simulink model "Robot_Project"  (R2025b)
settings: Solver=FixedStepDiscrete  StartTime=0.0  StopTime=10  FixedStep=0.01  RelTol=1e-3
model workspace (MAT data in the model file):
  Left_gain_calibration = 2.30921052632
  Right_gain_calibration = 1.47057847023
settings Model: Creator=Ahmed  LastModifiedBy=ENJAZ

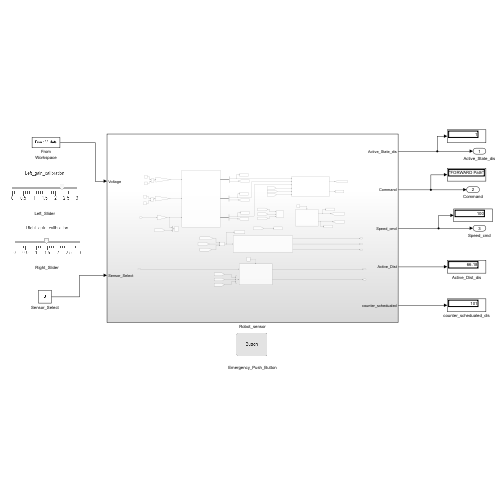
[thumbnail: Simulink's stored preview of the top-level diagram]
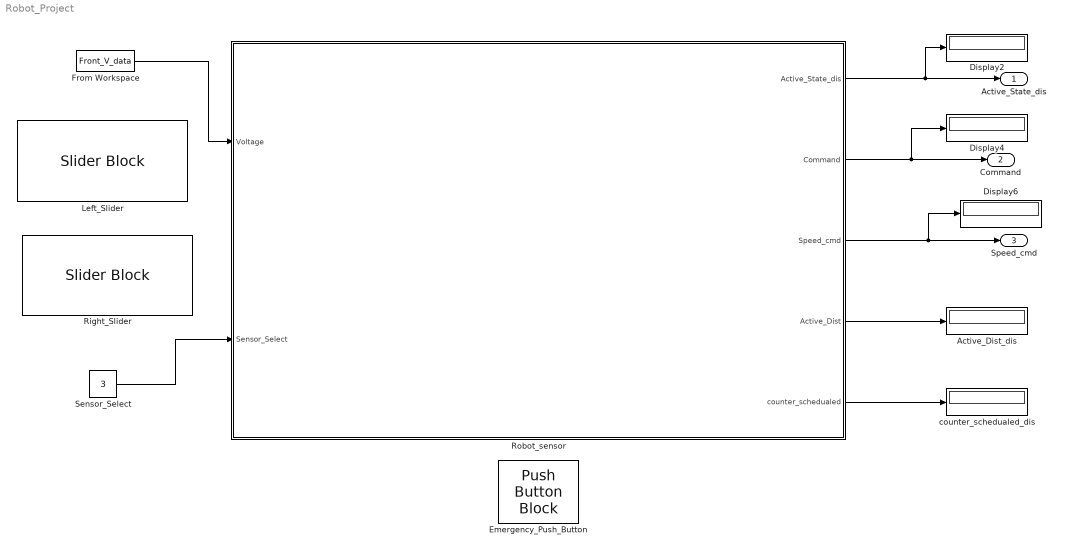
== system Robot_Project ==
  Active_Dist_dis : Display
  Display2 : Display
  Display4 : Display
  Display6 : Display
  Emergency_Push_Button : PushButtonBlock  ButtonType=Latch  IconOnColor=[0.0, 0.39215686274509803, 0.0]  IconOffColor=[0.0, 1.0, 0.0]  OffValue=0.000000
  From Workspace : FromWorkspace  VariableName=Front_V_data
  Left_Slider : SliderBlock  ScaleMax=3
  Right_Slider : SliderBlock  ScaleMax=3
  Robot_sensor : Subsystem
  Sensor_Select : Constant  Value=3
  counter_schedualed_dis : Display
  Active_State_dis : Outport
  Command : Outport  Port=2
  Speed_cmd : Outport  Port=3
  wires:
  Robot_sensor/2(Command) -> Command/1, Display4/1
  Robot_sensor/3(Speed_cmd) -> Display6/1, Speed_cmd/1
  From Workspace/1 -> Robot_sensor/1(Voltage)
  Sensor_Select/1 -> Robot_sensor/2(Sensor_Select)
  Robot_sensor/4(Active_Dist) -> Active_Dist_dis/1
  Robot_sensor/5(counter_schedualed) -> counter_schedualed_dis/1
  Robot_sensor/1(Active_State_dis) -> Active_State_dis/1, Display2/1

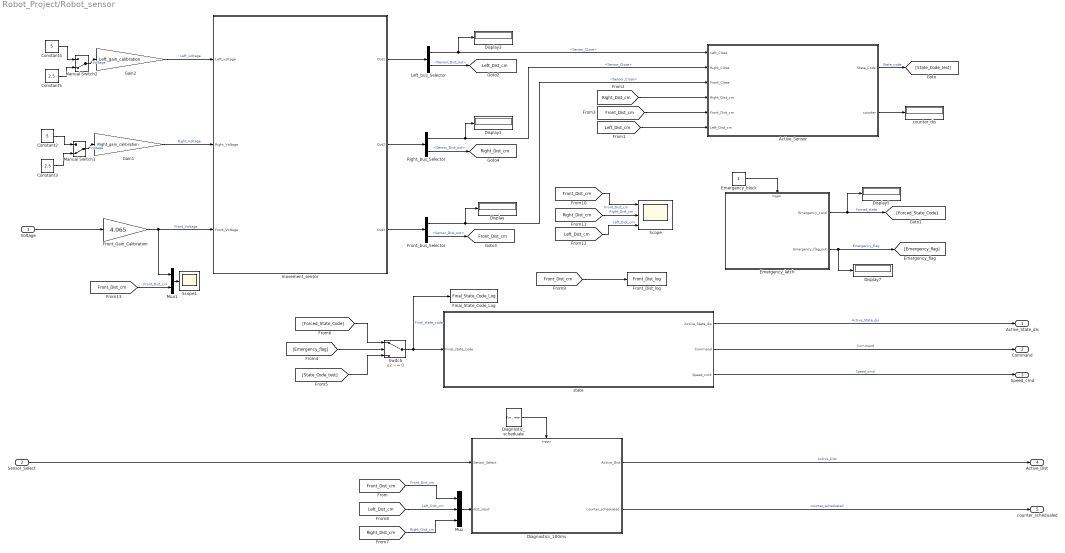
== system Robot_Project/Robot_sensor ==
  Voltage : Inport
  Sensor_Select : Inport  Port=2
  Active_Sensor : Subsystem
  Constant2 : Constant  Value=5
  Constant3 : Constant  Value=2.5
  Constant4 : Constant  Value=5
  Constant5 : Constant  Value=2.5
  Diagnostic_scheduale : FunctionCallGenerator  SampleTime=0.1
  Diagnostics_100ms : Subsystem  TreatAsAtomicUnit=on
  Display{,1,3,5,7} (5 alike) : Display
  Emergency_block : Constant
  Emergency_latch : Subsystem  TreatAsAtomicUnit=on
  Final_State_Code_Log : ToWorkspace  VariableName=Final_State_Code_Log  SaveFormat=Timeseries  SampleTime=-1
  Front_Dist_log : ToWorkspace  VariableName=Front_Dist_log  SaveFormat=Structure With Time  SampleTime=-1
  Front_Gain_Calibration : Gain  Gain=4.065
  Front_bus_Selector : BusSelector  OutputSignals=Sensor_Close,Sensor_Dist_out
  Gain1 : Gain  Gain=Right_gain_calibration
  Gain2 : Gain  Gain=Left_gain_calibration
  Left_bus_Selector : BusSelector  OutputSignals=Sensor_Close,Sensor_Dist_out
  Manual Switch1 : ManualSwitch  CurrentSetting=0
  Manual Switch2 : ManualSwitch  CurrentSetting=0
  Mux : Mux  Inputs=3
  Mux1 : Mux  Inputs=2
  Right_bus_Selector : BusSelector  OutputSignals=Sensor_Close,Sensor_Dist_out
  Scope : Scope  NumInputPorts=3
      settings: ActiveDisplayYMinimum=-1  ActiveDisplayYMaximum=1
  Scope1 : Scope
      settings: ActiveDisplayYMinimum=-43.187499999999993  ActiveDisplayYMaximum=393.6875
  Switch : Switch  Criteria=u2 ~= 0  SaturateOnIntegerOverflow=off  InputSameDT=off
  counter_dis : Display
  movement_sensor : Subsystem
  state : Subsystem
  Active_State_dis : Outport
  Command : Outport  Port=2
  Speed_cmd : Outport  Port=3
  Active_Dist : Outport  Port=4
  counter_schedualed : Outport  Port=5
  tag scope: Front_Dist_cm=global, Left_Dist_cm=global, Right_Dist_cm=global
  wires:
  Left_bus_Selector/1 -> Display3/1, Active_Sensor/1(Left_Close)  "<Sensor_Close>"
  state/1(Active_State_dis) -> Active_State_dis/1  "Active_State_dis"
  Manual Switch2/1 -> Gain2/1  "Voltage"
  Emergency_latch/1(Emergency_cond) -> Display5/1, [Forced_State_Code]  "forced_state"
  Manual Switch1/1 -> Gain1/1  "Voltage"
  [Right_Dist_cm] -> Mux/3  "Right_Dist_cm"
  Diagnostics_100ms/1(Active_Dist) -> Active_Dist/1  "Active_Dist"
  [Front_Dist_cm] -> Front_Dist_log/1
  Right_bus_Selector/1 -> Active_Sensor/2(Right_Close), Display1/1  "<Sensor_Close>"
  Diagnostic_scheduale/1 -> Diagnostics_100ms/Trigger
  [Front_Dist_cm] -> Active_Sensor/5(Front_Dist_cm)
  [State_Code_test] -> Switch/3
  Constant4/1 -> Manual Switch2/1
  [Forced_State_Code] -> Switch/1
  Front_Gain_Calibration/1 -> movement_sensor/3(Front_Voltage), Mux1/1  "Front_Voltage"
  state/2(Command) -> Command/1  "Command"
  Sensor_Select/1 -> Diagnostics_100ms/1(Sensor_Select)
  Front_bus_Selector/1 -> Active_Sensor/3(Front_Close), Display/1  "<Sensor_Close>"
  [Left_Dist_cm] -> Mux/2  "Left_Dist_cm"
  [Front_Dist_cm] -> Mux1/2  "Front_Dist_cm"
  Active_Sensor/1(State_Code) -> [State_Code_test]  "State_code"
  state/3(Speed_cmd) -> Speed_cmd/1  "Speed_cmd"
  Emergency_block/1 -> Emergency_latch/Trigger
  Constant2/1 -> Manual Switch1/1
  Mux/1 -> Diagnostics_100ms/2(dist_input)
  [Right_Dist_cm] -> Active_Sensor/4(Right_Dist_cm)
  [Emergency_flag] -> Switch/2
  Mux1/1 -> Scope1/1
  [Front_Dist_cm] -> Scope/1  "Front_Dist_cm"
  Left_bus_Selector/2 -> [Left_Dist_cm]  "<Sensor_Dist_out>"
  [Left_Dist_cm] -> Active_Sensor/6(Left_Dist_cm)
  [Left_Dist_cm] -> Scope/3  "Left_Dist_cm"
  Emergency_latch/2(Emergency_flag_out) -> Display7/1, [Emergency_flag]  "Emergency_flag"
  Switch/1 -> Final_State_Code_Log/1, state/1("Final_state_code ")  "Final_state_code"
  Diagnostics_100ms/2(counter_schedualed) -> counter_schedualed/1  "counter_schedualed"
  Constant3/1 -> Manual Switch1/2
  Constant5/1 -> Manual Switch2/2
  [Front_Dist_cm] -> Mux/1  "Front_Dist_cm"
  Front_bus_Selector/2 -> [Front_Dist_cm]  "<Sensor_Dist_out>"
  [Right_Dist_cm] -> Scope/2  "Right_Dist_cm"
  Right_bus_Selector/2 -> [Right_Dist_cm]  "<Sensor_Dist_out>"
  Voltage/1 -> Front_Gain_Calibration/1
  Gain2/1 -> movement_sensor/1(Left_voltage)  "Left_voltage"
  Gain1/1 -> movement_sensor/2(Right_Voltage)  "Right_Voltage"
  movement_sensor/1(Out1) -> Left_bus_Selector/1
  movement_sensor/2(Out2) -> Right_bus_Selector/1
  movement_sensor/3(Out3) -> Front_bus_Selector/1
  Active_Sensor/2(counter) -> counter_dis/1

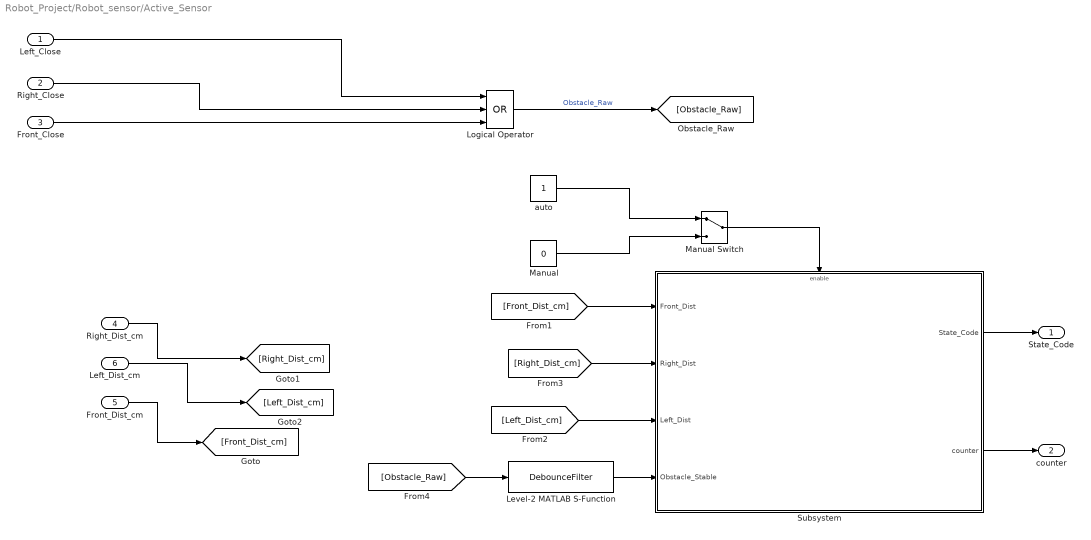
== system Robot_Project/Robot_sensor/Active_Sensor ==
  Left_Close : Inport
  Right_Close : Inport  Port=2
  Front_Close : Inport  Port=3
  Right_Dist_cm : Inport  Port=4
  Front_Dist_cm : Inport  Port=5
  Left_Dist_cm : Inport  Port=6
  Level-2 MATLAB S-Function : M-S-Function  FunctionName=DebounceFilter
  Logical Operator : Logic  Operator=OR  Inputs=3  AllPortsSameDT=off  OutDataTypeStr=boolean
  Manual : Constant  Value=0
  Manual Switch : ManualSwitch
  Subsystem : Subsystem
  auto : Constant
  State_Code : Outport
  counter : Outport  Port=2
  wires:
  Logical Operator/1 -> [Obstacle_Raw]  "Obstacle_Raw"
  Right_Close/1 -> Logical Operator/2
  Left_Close/1 -> Logical Operator/1
  Front_Close/1 -> Logical Operator/3
  Left_Dist_cm/1 -> [Left_Dist_cm]
  Right_Dist_cm/1 -> [Right_Dist_cm]
  Front_Dist_cm/1 -> [Front_Dist_cm]
  [Obstacle_Raw] -> Level-2 MATLAB S-Function/1
  [Front_Dist_cm] -> Subsystem/1(Front_Dist)
  [Right_Dist_cm] -> Subsystem/2(Right_Dist)
  [Left_Dist_cm] -> Subsystem/3(Left_Dist)
  Level-2 MATLAB S-Function/1 -> Subsystem/4(Obstacle_Stable)
  Subsystem/1(State_Code) -> State_Code/1
  auto/1 -> Manual Switch/1
  Manual Switch/1 -> Subsystem/Enable
  Manual/1 -> Manual Switch/2
  Subsystem/2(counter) -> counter/1

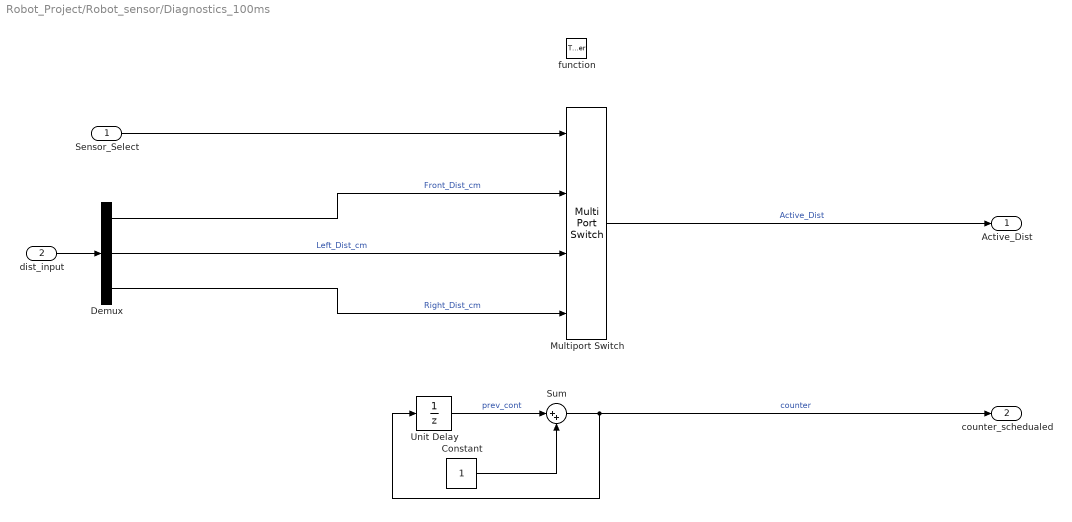
== system Robot_Project/Robot_sensor/Diagnostics_100ms ==
  Sensor_Select : Inport
  dist_input : Inport  Port=2
  function : TriggerPort  TriggerType=function-call  VariantControl=(inherit)
  Constant : Constant
  Demux : Demux  Outputs=3
  Multiport Switch : MultiPortSwitch  DiagnosticForDefault=None  SaturateOnIntegerOverflow=off  InputSameDT=off
  Sum : Sum  Inputs=|++
  Unit Delay : UnitDelay  SampleTime=-1  HasFrameUpgradeWarning=on
  Active_Dist : Outport
  counter_schedualed : Outport  Port=2
  wires:
  Constant/1 -> Sum/2
  Unit Delay/1 -> Sum/1  "prev_cont"
  Sum/1 -> Unit Delay/1, counter_schedualed/1  "counter"
  Demux/3 -> Multiport Switch/4  "Right_Dist_cm"
  Multiport Switch/1 -> Active_Dist/1  "Active_Dist"
  Demux/1 -> Multiport Switch/2  "Front_Dist_cm"
  Sensor_Select/1 -> Multiport Switch/1
  Demux/2 -> Multiport Switch/3  "Left_Dist_cm"
  dist_input/1 -> Demux/1

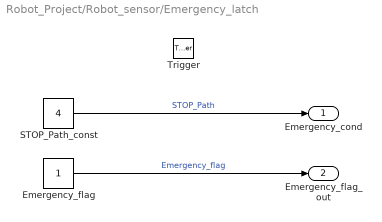
== system Robot_Project/Robot_sensor/Emergency_latch ==
  Trigger : TriggerPort  VariantControl=(inherit)
  Emergency_flag : Constant
  STOP_Path_const : Constant  Value=4
  Emergency_cond : Outport  InitialOutput=0
  Emergency_flag_out : Outport  Port=2  InitialOutput=0
  wires:
  STOP_Path_const/1 -> Emergency_cond/1  "STOP_Path"
  Emergency_flag/1 -> Emergency_flag_out/1  "Emergency_flag"

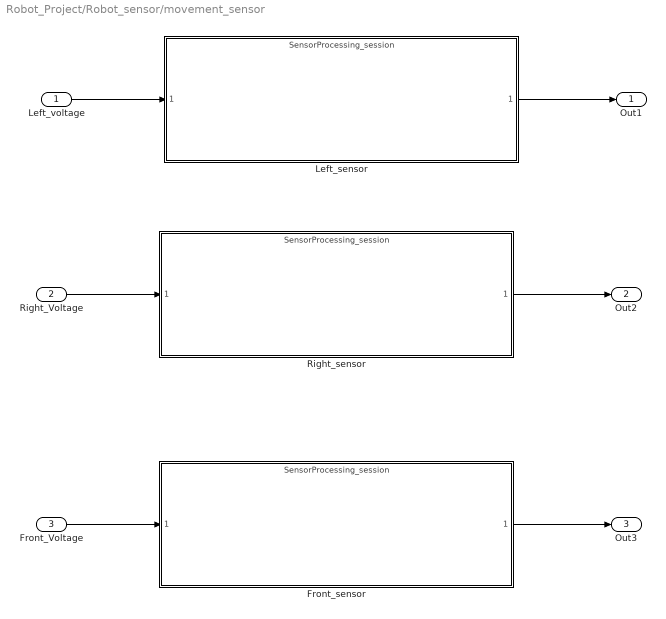
== system Robot_Project/Robot_sensor/movement_sensor ==
  Left_voltage : Inport
  Right_Voltage : Inport  Port=2
  Front_Voltage : Inport  Port=3
  Front_sensor : ModelReference  ModelNameDialog=SensorProcessing_session.slx  SimulationMode=Normal  ModelReferenceVersion=1.9
  Left_sensor : ModelReference  ModelNameDialog=SensorProcessing_session.slx  SimulationMode=Normal  ModelReferenceVersion=1.9
  Right_sensor : ModelReference  ModelNameDialog=SensorProcessing_session.slx  SimulationMode=Normal  ModelReferenceVersion=1.9
  Out1 : Outport
  Out2 : Outport  Port=2
  Out3 : Outport  Port=3
  wires:
  Right_sensor/1 -> Out2/1
  Left_sensor/1 -> Out1/1
  Front_sensor/1 -> Out3/1
  Left_voltage/1 -> Left_sensor/1
  Front_Voltage/1 -> Front_sensor/1
  Right_Voltage/1 -> Right_sensor/1

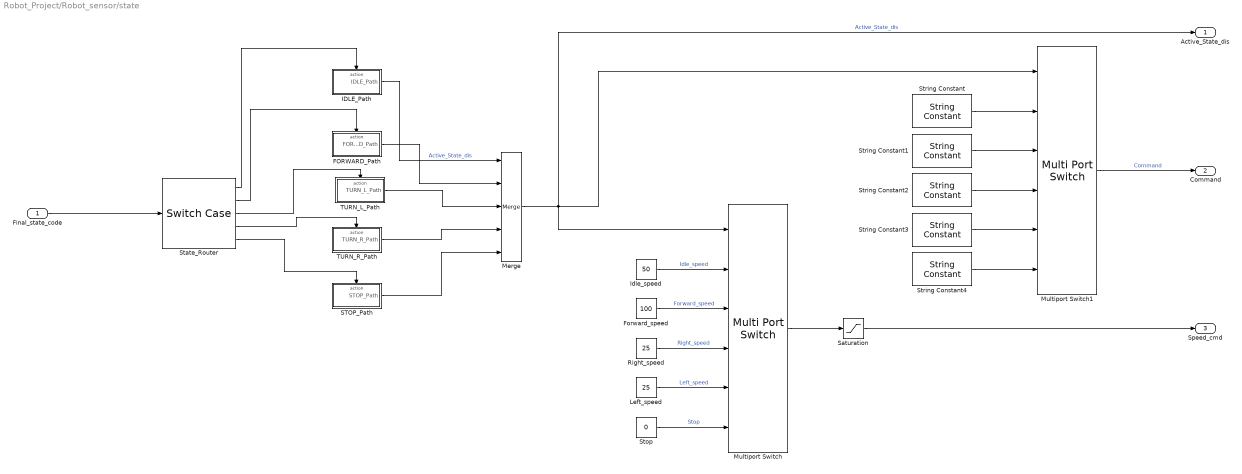
== system Robot_Project/Robot_sensor/state ==
  "Final_state_code " : Inport
  FORWARD_Path : Subsystem  TreatAsAtomicUnit=on
  Forward_speed : Constant  Value=100
  IDLE_Path : Subsystem  TreatAsAtomicUnit=on
  Idle_speed : Constant  Value=50
  Left_speed : Constant  Value=25
  Merge : Merge  Inputs=5
  Multiport Switch : MultiPortSwitch  DataPortOrder=Zero-based contiguous  Inputs=5  zeroidx=on  SaturateOnIntegerOverflow=off  InputSameDT=off
  Multiport Switch1 : MultiPortSwitch  DataPortOrder=Zero-based contiguous  Inputs=5  zeroidx=on  SaturateOnIntegerOverflow=off  InputSameDT=off
  Right_speed : Constant  Value=25
  STOP_Path : Subsystem  TreatAsAtomicUnit=on
  Saturation : Saturate  UpperLimit=100  LowerLimit=0
  State_Router : SwitchCase  CaseConditions={0,1,2,3,4}  ShowDefaultCase=off
  Stop : Constant  Value=0
  String Constant : StringConstant  String="\"IDLE Path\""
  String Constant1 : StringConstant  String="\"FORWARD Path\""
  String Constant2 : StringConstant  String="\"TURN Left\""
  String Constant3 : StringConstant  String="\"TURN Right\""
  String Constant4 : StringConstant  String="\"Stop\""
  TURN_L_Path : Subsystem  TreatAsAtomicUnit=on
  TURN_R_Path : Subsystem  TreatAsAtomicUnit=on
  Active_State_dis : Outport
  Command : Outport  Port=2
  Speed_cmd : Outport  Port=3
  wires:
  TURN_R_Path/1(TURN_R_Path) -> Merge/4
  State_Router/2 -> FORWARD_Path/Action
  STOP_Path/1(STOP_Path) -> Merge/5
  FORWARD_Path/1(FORWARD_Path) -> Merge/2
  TURN_L_Path/1(TURN_L_Path) -> Merge/3
  State_Router/4 -> TURN_R_Path/Action
  State_Router/1 -> IDLE_Path/Action
  State_Router/5 -> STOP_Path/Action
  State_Router/3 -> TURN_L_Path/Action
  Merge/1 -> Multiport Switch/1, Active_State_dis/1, Multiport Switch1/1  "Active_State_dis"
  "Final_state_code "/1 -> State_Router/1
  String Constant2/1 -> Multiport Switch1/4
  Multiport Switch1/1 -> Command/1  "Command"
  String Constant/1 -> Multiport Switch1/2
  String Constant3/1 -> Multiport Switch1/5
  String Constant1/1 -> Multiport Switch1/3
  String Constant4/1 -> Multiport Switch1/6
  Saturation/1 -> Speed_cmd/1
  Right_speed/1 -> Multiport Switch/4  "Right_speed"
  Forward_speed/1 -> Multiport Switch/3  "Forward_speed"
  Left_speed/1 -> Multiport Switch/5  "Left_speed"
  Stop/1 -> Multiport Switch/6  "Stop"
  Idle_speed/1 -> Multiport Switch/2  "Idle_speed"
  Multiport Switch/1 -> Saturation/1
  IDLE_Path/1(IDLE_Path) -> Merge/1  "Active_State_dis"

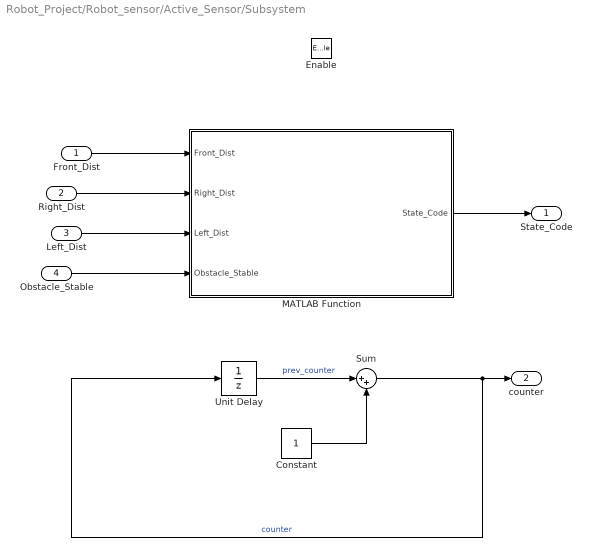
== system Robot_Project/Robot_sensor/Active_Sensor/Subsystem ==
  Front_Dist : Inport
  Right_Dist : Inport  Port=2
  Left_Dist : Inport  Port=3
  Obstacle_Stable : Inport  Port=4
  Enable : EnablePort
  Constant : Constant
  MATLAB Function : MATLAB Function  TreatAsAtomicUnit=on
  Sum : Sum  Inputs=|++
  Unit Delay : UnitDelay  SampleTime=-1  HasFrameUpgradeWarning=on
  State_Code : Outport
  counter : Outport  Port=2
  wires:
  MATLAB Function/1(State_Code) -> State_Code/1
  Obstacle_Stable/1 -> MATLAB Function/4(Obstacle_Stable)
  Front_Dist/1 -> MATLAB Function/1(Front_Dist)
  Right_Dist/1 -> MATLAB Function/2(Right_Dist)
  Left_Dist/1 -> MATLAB Function/3(Left_Dist)
  Sum/1 -> Unit Delay/1, counter/1  "counter"
  Constant/1 -> Sum/2
  Unit Delay/1 -> Sum/1  "prev_counter"

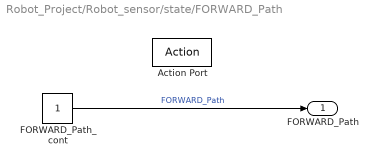
== system Robot_Project/Robot_sensor/state/FORWARD_Path ==
  Action Port : ActionPort  ActionPortLabel=case [ 1 ]:
  FORWARD_Path_cont : Constant
  FORWARD_Path : Outport
  wires:
  FORWARD_Path_cont/1 -> FORWARD_Path/1  "FORWARD_Path"

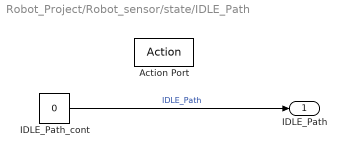
== system Robot_Project/Robot_sensor/state/IDLE_Path ==
  Action Port : ActionPort  ActionPortLabel=case [ 0 ]:
  IDLE_Path_cont : Constant  Value=0
  IDLE_Path : Outport
  wires:
  IDLE_Path_cont/1 -> IDLE_Path/1  "IDLE_Path"

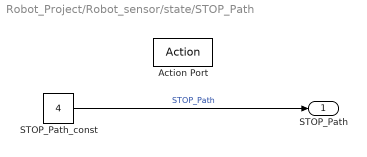
== system Robot_Project/Robot_sensor/state/STOP_Path ==
  Action Port : ActionPort  ActionPortLabel=case [ 4 ]:
  STOP_Path_const : Constant  Value=4
  STOP_Path : Outport
  wires:
  STOP_Path_const/1 -> STOP_Path/1  "STOP_Path"

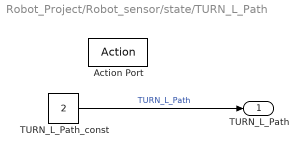
== system Robot_Project/Robot_sensor/state/TURN_L_Path ==
  Action Port : ActionPort  ActionPortLabel=case [ 2 ]:
  TURN_L_Path_const : Constant  Value=2
  TURN_L_Path : Outport
  wires:
  TURN_L_Path_const/1 -> TURN_L_Path/1  "TURN_L_Path"

== system Robot_Project/Robot_sensor/state/TURN_R_Path ==
  Action Port : ActionPort  ActionPortLabel=case [ 3 ]:
  TURN_R_Path_const : Constant  Value=3
  TURN_R_Path : Outport
  wires:
  TURN_R_Path_const/1 -> TURN_R_Path/1  "TURN_R_Path"

== matlab function Robot_Project/Robot_sensor/Active_Sensor/Subsystem/MATLAB Function ==
  data: Front_Dist input; State_Code output; Right_Dist input; Left_Dist input; Obstacle_Stable input
function State_Code  = DecideRobotState(Front_Dist, Right_Dist, Left_Dist, Obstacle_Stable)

    if Obstacle_Stable && Front_Dist < 20
        State_Code = int32(4);
    elseif Obstacle_Stable && Front_Dist < 40 && Left_Dist > Right_Dist
        State_Code = int32(2);
    elseif Obstacle_Stable && Front_Dist < 40
        State_Code = int32(3);
    elseif Front_Dist >= 40
        State_Code = int32(1);
    else
        State_Code = int32(0);
    end
    
end
